simulink model "Discrete_Closed_Loop_Model_74_prelude_simu"  (Simulink 7.8)
settings: Solver=FixedStepDiscrete  StartTime=0.0  StopTime=0.5  FixedStep=dt  RelTol=1e-3
values from neighbouring files (symbols this model uses):
  hc = u(2,k)    [Simul_modele.m]    (also in Simul_modele2.m; Simul_modele3.m; Simul_modele4.m; Simul_modele5.m)
  hcInit = 1e4    (= 10000)    [Simul_modele6.m]    (also in Simul_modele8.m)
  S = sortrows([V' diag(D)],3)    [drawEllipse.m]    (also in tarbouriech04_discret.m = sdpvar(m,m,'diagonal'); tarbouriech05_continu.m = sdpvar(m,m,'diagonal'))
undefined symbols (not defined in the file or in its folder): A_de, A_dx, alpha_0, Az_az, Az_h, Az_q, Az_Va, Az_Vz, B_de, B_dx, Bz_az, Bz_h, Bz_q, Bz_Va, Bz_Vz, C_de, C_dx, cbar, CD_0, CD_alpha, CD_deltae, CI_AltHold, CI_de, CI_dx, CI_FD, CIz_az, CIz_h, CIz_q, CIz_Va, CIz_Vz, CL_alpha, CL_deltae, Cm_0, Cm_alpha, Cm_deltae, Cm_q, Cz_az, Cz_h, Cz_q, Cz_Va, Cz_Vz, D_de, D_dx, delta_e_eq, delta_x_eq, DiscIntNeverNeededParam, dt_dx, Dz_az, Dz_h, Dz_q, Dz_Va, Dz_Vz, g0, h_eq, I_y, K1_intVa, K1_q, K1_Va, K1_Vz, K2_az ... (+21)
settings Model: Creator=David  LastModifiedBy=rpichard  ExtModeAutoUpdateStatusClock=off
settings DataIOCC: LimitDataPoints=off
settings DebuggingCC: SaveWithParameterizedLinksMsg=none  MultiTaskDSMMsg=warning  MultiTaskCondExecSysMsg=none
settings HardwareCC: TargetHWDeviceType=32-bit Generic
settings SFSimCC: SimParseCustomCode=off
settings RTWCC: IncludeERTFirstTime=on
settings CodeAppCC: CustomSymbolStrType=$N$R$M_T
settings GRTTargetCC: TargetFcnLib=ansi_tfl_tmw.mat

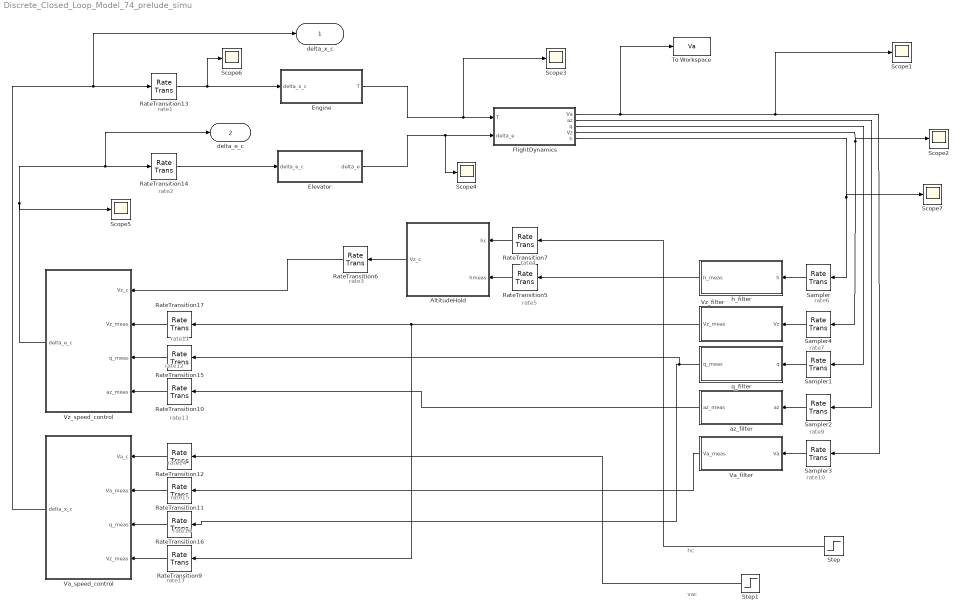
== system Discrete_Closed_Loop_Model_74_prelude_simu ==
  note: rate1
  note: rate2
  note: rate3
  note: rate4
  note: rate5
  note: rate6
  note: rate7
  note: rate9
  note: rate10
  note: rate11
  note: rate12
  note: rate13
  note: rate14
  note: rate15
  note: rate16
  note: rate17
  note: hc
  note: vac
  "AltitudeHold  " : Subsystem
  Elevator : Subsystem
  Engine : Subsystem
  FlightDynamics : Subsystem
  RateTransition{6,10,15,17} (4 alike) : RateTransition  OutPortSampleTime=Ts_K2
  RateTransition{9,11..12,16} (4 alike) : RateTransition  OutPortSampleTime=Ts_K1
  RateTransition13 : RateTransition  X0=delta_x_eq  OutPortSampleTime=dt_dx
  RateTransition14 : RateTransition  X0=delta_e_eq  OutPortSampleTime=dt_de
  RateTransition5 : RateTransition  X0=h_eq  OutPortSampleTime=Ts_h
  RateTransition7 : RateTransition  OutPortSampleTime=Ts_h
  Sampler : RateTransition  X0=h_eq  OutPortSampleTime=Ts_f_h
  Sampler1 : RateTransition  OutPortSampleTime=Ts_f_q
  Sampler2 : RateTransition  OutPortSampleTime=Ts_f_az
  Sampler3 : RateTransition  X0=Va_eq  OutPortSampleTime=Ts_f_Va
      settings: AttributesFormatString=%<Name>
  Sampler4 : RateTransition  OutPortSampleTime=Ts_f_Vz
  Scope{1..7} (7 alike) : Scope
      Scope1 settings: SaveName=ScopeData2
      Scope2 settings: SaveName=ScopeData4
      Scope3 settings: SaveName=ScopeData6
      Scope4 settings: SaveName=ScopeData7
      Scope5 settings: SaveName=ScopeData9
      Scope6 settings: SaveName=ScopeData10
      Scope7 settings: YMin=9990  YMax=10210  SaveName=ScopeData11
  Step : Step  Time=0  Before=hcInit  After=hc  SampleTime=0
  Step1 : Step  Before=235  After=235  SampleTime=0
  To Workspace : ToWorkspace  VariableName=Va  SampleTime=-1  SaveFormat=Array
  Va_filter : Subsystem
  Va_speed_control : Subsystem
  "Vz_filter " : Subsystem
  Vz_speed_control : Subsystem
  az_filter : Subsystem
  "h_filter " : Subsystem
  q_filter : Subsystem
  delta_x_c : Outport
  delta_e_c : Outport  Port=2
  wires:
  Step1/1 -> RateTransition12/1
  FlightDynamics/1(Va) -> Sampler3/1, Scope1/1, To Workspace/1
  FlightDynamics/2(az) -> Sampler2/1
  FlightDynamics/3(q) -> Sampler1/1
  FlightDynamics/4(Vz) -> Sampler4/1, Scope2/1
  Engine/1(T) -> FlightDynamics/1(T), Scope3/1
  Elevator/1(delta_e) -> FlightDynamics/2(delta_e), Scope4/1
  Va_filter/1(Va_meas) -> RateTransition11/1
  "AltitudeHold  "/1(Vz_c) -> RateTransition6/1
  Step/1 -> RateTransition7/1
  FlightDynamics/5(h) -> Sampler/1, Scope7/1
  az_filter/1(az_meas) -> RateTransition10/1
  RateTransition7/1 -> "AltitudeHold  "/1(hc)
  q_filter/1(q_meas) -> RateTransition15/1, RateTransition16/1
  RateTransition10/1 -> Vz_speed_control/4(az_meas)
  RateTransition11/1 -> Va_speed_control/2(Va_meas)
  RateTransition12/1 -> Va_speed_control/1(Va_c)
  Vz_speed_control/1(delta_e_c) -> RateTransition14/1, delta_e_c/1, Scope5/1
  Va_speed_control/1(delta_x_c) -> RateTransition13/1, delta_x_c/1
  RateTransition13/1 -> Engine/1(delta_x_c), Scope6/1
  "h_filter "/1(h_meas) -> RateTransition5/1
  RateTransition15/1 -> Vz_speed_control/3(q_meas)
  RateTransition16/1 -> Va_speed_control/3(q_meas)
  "Vz_filter "/1(Vz_meas) -> RateTransition17/1, RateTransition9/1
  RateTransition9/1 -> Va_speed_control/4(Vz_meas)
  Sampler/1 -> "h_filter "/1(h)
  Sampler4/1 -> "Vz_filter "/1(Vz)
  Sampler1/1 -> q_filter/1(q)
  Sampler2/1 -> az_filter/1(az)
  Sampler3/1 -> Va_filter/1(Va)
  RateTransition5/1 -> "AltitudeHold  "/2(hmeas)
  RateTransition17/1 -> Vz_speed_control/2(Vz_meas)
  RateTransition6/1 -> Vz_speed_control/1(Vz_c)
  RateTransition14/1 -> Elevator/1(delta_e_c)

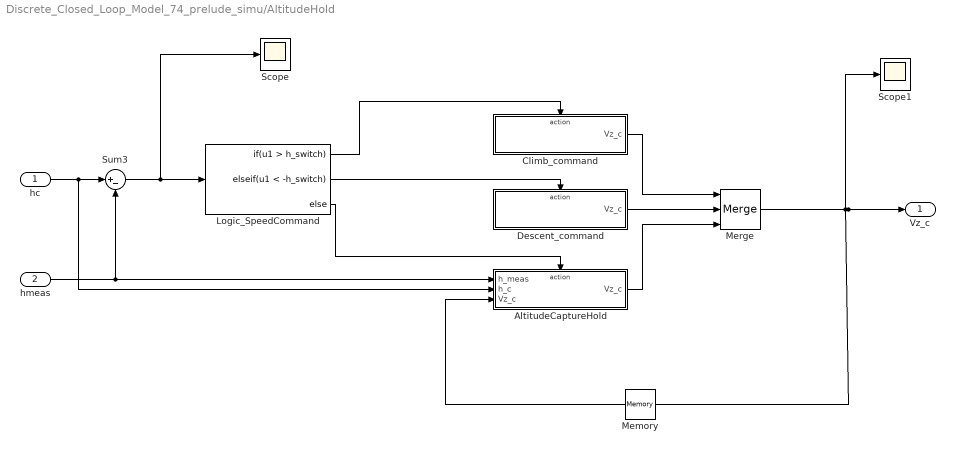
== system Discrete_Closed_Loop_Model_74_prelude_simu/AltitudeHold   ==
  hc : Inport
  hmeas : Inport  Port=2
  AltitudeCaptureHold : Subsystem  TreatAsAtomicUnit=on
  Climb_command : Subsystem  TreatAsAtomicUnit=on
  Descent_command : Subsystem  TreatAsAtomicUnit=on
  Logic_SpeedCommand : If  IfExpression=u1 > h_switch  ElseIfExpressions=u1 < -h_switch
  Memory : Memory  InheritSampleTime=on
  Merge : Merge  Inputs=3
  Scope : Scope
  Scope1 : Scope
      settings: SaveName=ScopeData12
  Sum3 : Sum  Inputs=|+-  SampleTime=Ts_h  OutDataTypeStr=Inherit: Same as first input
  Vz_c : Outport
  wires:
  hc/1 -> AltitudeCaptureHold/2(h_c), Sum3/1
  hmeas/1 -> Sum3/2, AltitudeCaptureHold/1(h_meas)
  Sum3/1 -> Logic_SpeedCommand/1, Scope/1
  Logic_SpeedCommand/1 -> Climb_command/Action
  Logic_SpeedCommand/3 -> AltitudeCaptureHold/Action
  Logic_SpeedCommand/2 -> Descent_command/Action
  Descent_command/1(Vz_c) -> Merge/2
  Climb_command/1(Vz_c) -> Merge/1
  AltitudeCaptureHold/1("Vz_c ") -> Merge/3
  Merge/1 -> Vz_c/1, Memory/1, Scope1/1
  Memory/1 -> AltitudeCaptureHold/3(Vz_c)

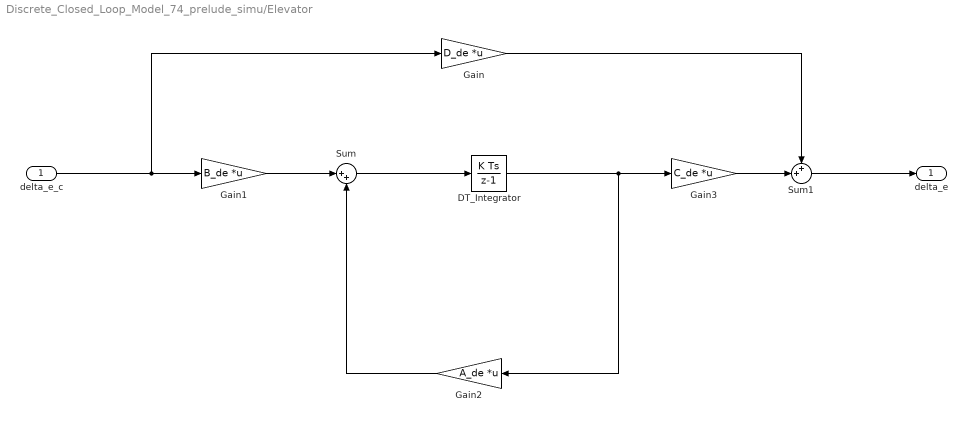
== system Discrete_Closed_Loop_Model_74_prelude_simu/Elevator ==
  delta_e_c : Inport
  DT_Integrator : DiscreteIntegrator  InitialCondition=CI_de  SampleTime=dt_dx  ICPrevOutput=DiscIntNeverNeededParam  ICPrevScaledInput=DiscIntNeverNeededParam
  Gain : Gain  Gain=D_de  Multiplication=Matrix(K*u)  OutDataTypeStr=Inherit: Same as input  ParamDataTypeStr=Inherit: Same as input
  Gain1 : Gain  Gain=B_de  Multiplication=Matrix(K*u)  OutDataTypeStr=Inherit: Same as input  ParamDataTypeStr=Inherit: Same as input
  Gain2 : Gain  Gain=A_de  Multiplication=Matrix(K*u)  OutDataTypeStr=Inherit: Same as input  ParamDataTypeStr=Inherit: Same as input
  Gain3 : Gain  Gain=C_de  Multiplication=Matrix(K*u)  OutDataTypeStr=Inherit: Same as input  ParamDataTypeStr=Inherit: Same as input
  Sum : Sum  Inputs=|++  OutDataTypeStr=Inherit: Same as first input
  Sum1 : Sum  Inputs=++|  OutDataTypeStr=Inherit: Same as first input
  delta_e : Outport
  wires:
  delta_e_c/1 -> Gain/1, Gain1/1
  Sum1/1 -> delta_e/1
  Sum/1 -> DT_Integrator/1
  Gain/1 -> Sum1/1
  Gain1/1 -> Sum/1
  Gain2/1 -> Sum/2
  Gain3/1 -> Sum1/2
  DT_Integrator/1 -> Gain2/1, Gain3/1

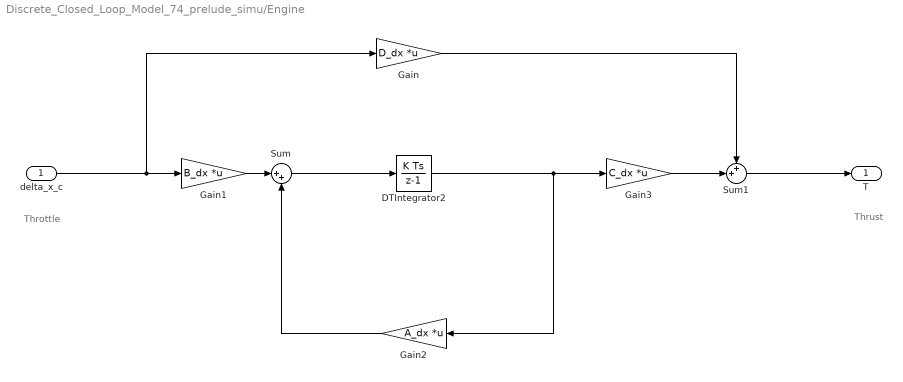
== system Discrete_Closed_Loop_Model_74_prelude_simu/Engine ==
  note: Throttle
  note: Thrust
  delta_x_c : Inport
  DTIntegrator2 : DiscreteIntegrator  InitialCondition=CI_dx  SampleTime=dt_dx  ICPrevOutput=DiscIntNeverNeededParam  ICPrevScaledInput=DiscIntNeverNeededParam
  Gain : Gain  Gain=D_dx  Multiplication=Matrix(K*u)  OutDataTypeStr=Inherit: Same as input  ParamDataTypeStr=Inherit: Same as input
  Gain1 : Gain  Gain=B_dx  Multiplication=Matrix(K*u)  OutDataTypeStr=Inherit: Same as input  ParamDataTypeStr=Inherit: Same as input
  Gain2 : Gain  Gain=A_dx  Multiplication=Matrix(K*u)  OutDataTypeStr=Inherit: Same as input  ParamDataTypeStr=Inherit: Same as input
  Gain3 : Gain  Gain=C_dx  Multiplication=Matrix(K*u)  OutDataTypeStr=Inherit: Same as input  ParamDataTypeStr=Inherit: Same as input
  Sum : Sum  Inputs=|++  OutDataTypeStr=Inherit: Same as first input
  Sum1 : Sum  Inputs=++|  OutDataTypeStr=Inherit: Same as first input
  T : Outport
  wires:
  delta_x_c/1 -> Gain/1, Gain1/1
  Sum1/1 -> T/1
  DTIntegrator2/1 -> Gain2/1, Gain3/1
  Sum/1 -> DTIntegrator2/1
  Gain/1 -> Sum1/1
  Gain1/1 -> Sum/1
  Gain2/1 -> Sum/2
  Gain3/1 -> Sum1/2

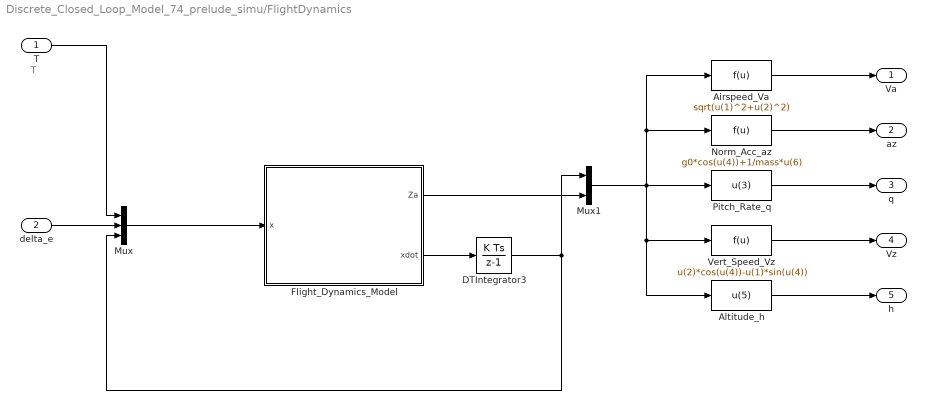
== system Discrete_Closed_Loop_Model_74_prelude_simu/FlightDynamics ==
  note: T
  T : Inport
  delta_e : Inport  Port=2
  "Airspeed_Va  " : Fcn  Expr=sqrt(u(1)^2+u(2)^2)
  Altitude_h : Fcn  Expr=u(5)
  DTIntegrator3 : DiscreteIntegrator  InitialCondition=CI_FD  SampleTime=dt_dx  ICPrevOutput=DiscIntNeverNeededParam  ICPrevScaledInput=DiscIntNeverNeededParam
  Flight_Dynamics_Model : Subsystem
  Mux : Mux  Inputs=3
  Mux1 : Mux  Inputs=2
  "Norm_Acc_az  " : Fcn  Expr=g0*cos(u(4))+1/mass*u(6)
  "Pitch_Rate_q " : Fcn  Expr=u(3)
  Vert_Speed_Vz : Fcn  Expr=u(2)*cos(u(4))-u(1)*sin(u(4))
  Va : Outport
  az : Outport  Port=2
  q : Outport  Port=3
  Vz : Outport  Port=4
  h : Outport  Port=5
  wires:
  delta_e/1 -> Mux/2
  DTIntegrator3/1 -> Mux/3, Mux1/1
  T/1 -> Mux/1
  Mux/1 -> Flight_Dynamics_Model/1(x)
  Flight_Dynamics_Model/2(xdot) -> DTIntegrator3/1
  Altitude_h/1 -> h/1
  Vert_Speed_Vz/1 -> Vz/1
  "Pitch_Rate_q "/1 -> q/1
  "Norm_Acc_az  "/1 -> az/1
  "Airspeed_Va  "/1 -> Va/1
  Flight_Dynamics_Model/1(Za) -> Mux1/2
  Mux1/1 -> "Pitch_Rate_q "/1, "Norm_Acc_az  "/1, "Airspeed_Va  "/1, Vert_Speed_Vz/1, Altitude_h/1

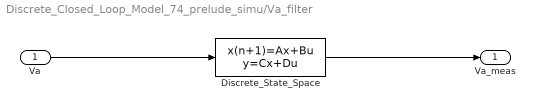
== system Discrete_Closed_Loop_Model_74_prelude_simu/Va_filter ==
  Va : Inport
  Discrete_State_Space : DiscreteStateSpace  A=Az_Va  B=Bz_Va  C=Cz_Va  D=Dz_Va  X0=CIz_Va  SampleTime=Ts_f_Va
  Va_meas : Outport
  wires:
  Discrete_State_Space/1 -> Va_meas/1
  Va/1 -> Discrete_State_Space/1

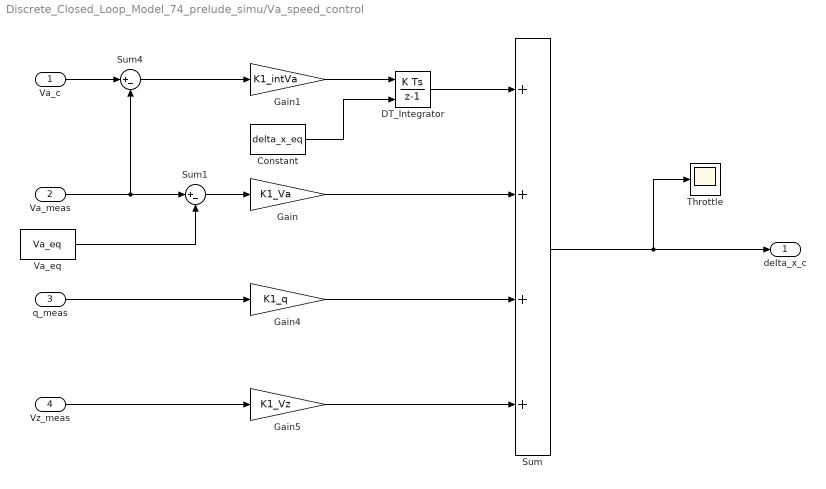
== system Discrete_Closed_Loop_Model_74_prelude_simu/Va_speed_control ==
  Va_c : Inport
  Va_meas : Inport  Port=2
  q_meas : Inport  Port=3
  Vz_meas : Inport  Port=4
  Constant : Constant  Value=delta_x_eq  SampleTime=Ts_K1
  DT_Integrator : DiscreteIntegrator  InitialConditionSource=external  SampleTime=Ts_K1  ICPrevOutput=DiscIntNeverNeededParam  ICPrevScaledInput=DiscIntNeverNeededParam
  Gain : Gain  Gain=K1_Va  OutDataTypeStr=Inherit: Same as input  ParamDataTypeStr=Inherit: Same as input
  Gain1 : Gain  Gain=K1_intVa  OutDataTypeStr=Inherit: Same as input  ParamDataTypeStr=Inherit: Same as input
  Gain4 : Gain  Gain=K1_q  OutDataTypeStr=Inherit: Same as input  ParamDataTypeStr=Inherit: Same as input
  Gain5 : Gain  Gain=K1_Vz  OutDataTypeStr=Inherit: Same as input  ParamDataTypeStr=Inherit: Same as input
  Sum : Sum  Inputs=++++  SampleTime=Ts_K1  OutDataTypeStr=Inherit: Same as first input
  Sum1 : Sum  Inputs=|+-  SampleTime=Ts_K1  OutDataTypeStr=Inherit: Same as first input
  Sum4 : Sum  Inputs=|+-  SampleTime=Ts_K1  OutDataTypeStr=Inherit: Same as first input
  Throttle : Scope
      settings: YMin=10094  YMax=10100.5  SaveName=ScopeData5  DataFormat=Array
  Va_eq : Constant  Value=Va_eq  SampleTime=Ts_K1
  delta_x_c : Outport
  wires:
  Va_meas/1 -> Sum1/1, Sum4/2
  Sum1/1 -> Gain/1
  Gain/1 -> Sum/2
  Va_c/1 -> Sum4/1
  Gain1/1 -> DT_Integrator/1
  q_meas/1 -> Gain4/1
  Vz_meas/1 -> Gain5/1
  Gain4/1 -> Sum/3
  Gain5/1 -> Sum/4
  Sum/1 -> Throttle/1, delta_x_c/1
  Constant/1 -> DT_Integrator/2
  Va_eq/1 -> Sum1/2
  Sum4/1 -> Gain1/1
  DT_Integrator/1 -> Sum/1

== system Discrete_Closed_Loop_Model_74_prelude_simu/Vz_filter  ==
  Vz : Inport
  Discrete_State_Space : DiscreteStateSpace  A=Az_Vz  B=Bz_Vz  C=Cz_Vz  D=Dz_Vz  X0=CIz_Vz  SampleTime=Ts_f_Vz
  Vz_meas : Outport
  wires:
  Discrete_State_Space/1 -> Vz_meas/1
  Vz/1 -> Discrete_State_Space/1

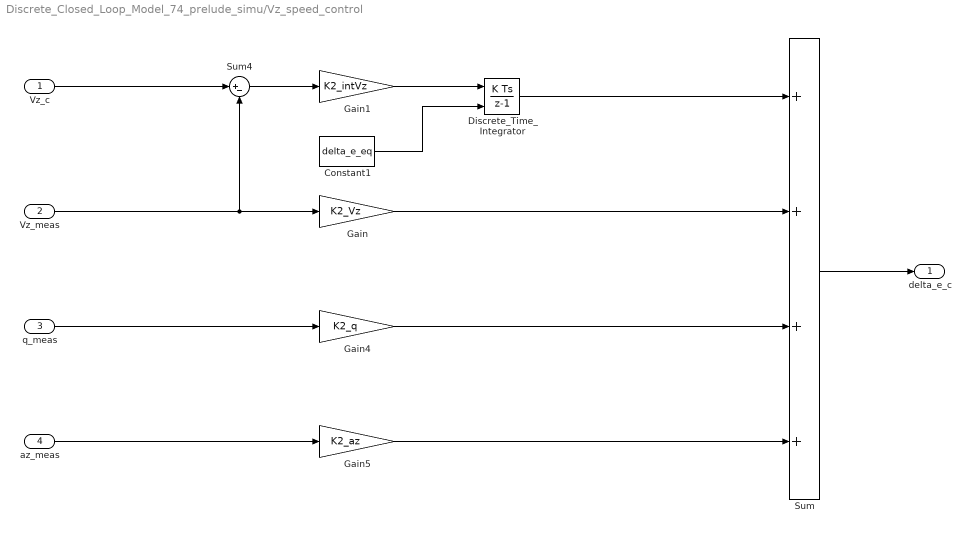
== system Discrete_Closed_Loop_Model_74_prelude_simu/Vz_speed_control ==
  Vz_c : Inport
  Vz_meas : Inport  Port=2
  q_meas : Inport  Port=3
  az_meas : Inport  Port=4
  Constant1 : Constant  Value=delta_e_eq  SampleTime=Ts_K2
  Discrete_Time_Integrator : DiscreteIntegrator  InitialConditionSource=external  SampleTime=Ts_K2  ICPrevOutput=DiscIntNeverNeededParam  ICPrevScaledInput=DiscIntNeverNeededParam
  Gain : Gain  Gain=K2_Vz  OutDataTypeStr=Inherit: Same as input  ParamDataTypeStr=Inherit: Same as input
  Gain1 : Gain  Gain=K2_intVz  OutDataTypeStr=Inherit: Same as input  ParamDataTypeStr=Inherit: Same as input
  Gain4 : Gain  Gain=K2_q  OutDataTypeStr=Inherit: Same as input  ParamDataTypeStr=Inherit: Same as input
  Gain5 : Gain  Gain=K2_az  OutDataTypeStr=Inherit: Same as input  ParamDataTypeStr=Inherit: Same as input
  Sum : Sum  Inputs=++++  SampleTime=Ts_K2  OutDataTypeStr=Inherit: Same as first input
  Sum4 : Sum  Inputs=|+-  OutDataTypeStr=Inherit: Same as first input
  delta_e_c : Outport
  wires:
  Vz_meas/1 -> Sum4/2, Gain/1
  Gain/1 -> Sum/2
  Vz_c/1 -> Sum4/1
  Gain1/1 -> Discrete_Time_Integrator/1
  q_meas/1 -> Gain4/1
  az_meas/1 -> Gain5/1
  Gain4/1 -> Sum/3
  Gain5/1 -> Sum/4
  Sum/1 -> delta_e_c/1
  Sum4/1 -> Gain1/1
  Discrete_Time_Integrator/1 -> Sum/1
  Constant1/1 -> Discrete_Time_Integrator/2

== system Discrete_Closed_Loop_Model_74_prelude_simu/az_filter ==
  az : Inport
  Discrete_State_Space : DiscreteStateSpace  A=Az_az  B=Bz_az  C=Cz_az  D=Dz_az  X0=CIz_az  SampleTime=Ts_f_az
  az_meas : Outport
  wires:
  Discrete_State_Space/1 -> az_meas/1
  az/1 -> Discrete_State_Space/1

== system Discrete_Closed_Loop_Model_74_prelude_simu/h_filter  ==
  h : Inport
  Discrete_State_Space : DiscreteStateSpace  A=Az_h  B=Bz_h  C=Cz_h  D=Dz_h  X0=CIz_h  SampleTime=Ts_f_h
  h_meas : Outport
  wires:
  Discrete_State_Space/1 -> h_meas/1
  h/1 -> Discrete_State_Space/1

== system Discrete_Closed_Loop_Model_74_prelude_simu/q_filter ==
  q : Inport
  Discrete_State_Space : DiscreteStateSpace  A=Az_q  B=Bz_q  C=Cz_q  D=Dz_q  X0=CIz_q  SampleTime=Ts_f_q
  q_meas : Outport
  wires:
  Discrete_State_Space/1 -> q_meas/1
  q/1 -> Discrete_State_Space/1

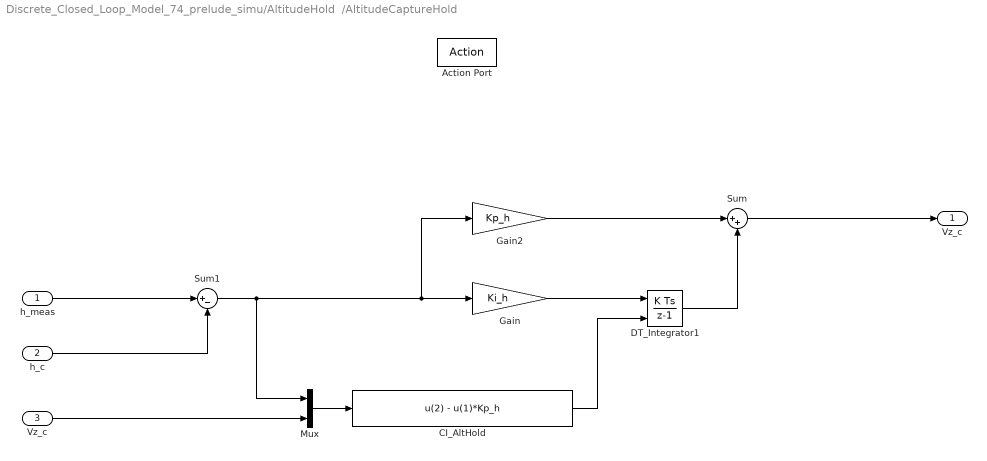
== system Discrete_Closed_Loop_Model_74_prelude_simu/AltitudeHold  /AltitudeCaptureHold ==
  h_meas : Inport
  h_c : Inport  Port=2
  Vz_c : Inport  Port=3
  Action Port : ActionPort  InitializeStates=reset  ActionType=else
  CI_AltHold : Fcn  Expr=u(2) - u(1)*Kp_h
  DT_Integrator1 : DiscreteIntegrator  InitialConditionSource=external  InitialCondition=CI_AltHold  SampleTime=Ts_h  ICPrevOutput=DiscIntNeverNeededParam  ICPrevScaledInput=DiscIntNeverNeededParam
  Gain : Gain  Gain=Ki_h  OutDataTypeStr=Inherit: Same as input  ParamDataTypeStr=Inherit: Same as input
  Gain2 : Gain  Gain=Kp_h  OutDataTypeStr=Inherit: Same as input  ParamDataTypeStr=Inherit: Same as input
  Mux : Mux  Inputs=2
  Sum : Sum  Inputs=|++  OutDataTypeStr=Inherit: Same as first input
  Sum1 : Sum  Inputs=|+-  OutDataTypeStr=Inherit: Same as first input
  "Vz_c " : Outport
  wires:
  Gain/1 -> DT_Integrator1/1
  Gain2/1 -> Sum/1
  h_meas/1 -> Sum1/1
  CI_AltHold/1 -> DT_Integrator1/2
  Sum/1 -> "Vz_c "/1
  Sum1/1 -> Mux/1, Gain/1, Gain2/1
  h_c/1 -> Sum1/2
  DT_Integrator1/1 -> Sum/2
  Mux/1 -> CI_AltHold/1
  Vz_c/1 -> Mux/2

== system Discrete_Closed_Loop_Model_74_prelude_simu/AltitudeHold  /Climb_command ==
  Action Port : ActionPort  ActionType=then
  h_switch2 : Constant  Value=Vz_c  SampleTime=Ts_h
  Vz_c : Outport
  wires:
  h_switch2/1 -> Vz_c/1

== system Discrete_Closed_Loop_Model_74_prelude_simu/AltitudeHold  /Descent_command ==
  Action Port : ActionPort  InitializeStates=reset  ActionType=elseif
  h_switch4 : Constant  Value=-Vz_c  SampleTime=Ts_h
  Vz_c : Outport
  wires:
  h_switch4/1 -> Vz_c/1

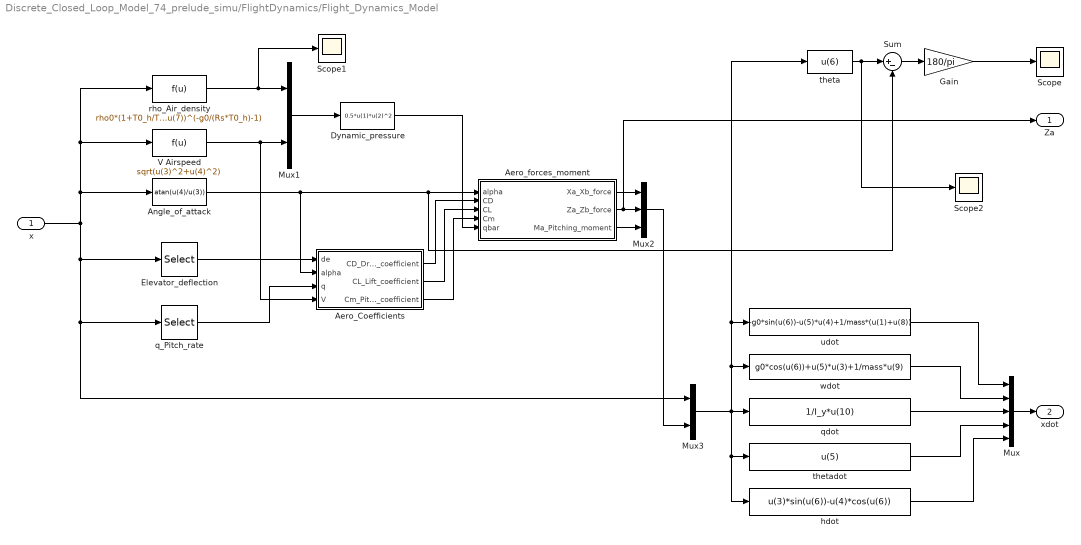
== system Discrete_Closed_Loop_Model_74_prelude_simu/FlightDynamics/Flight_Dynamics_Model ==
  x : Inport
  Aero_Coefficients : Subsystem
  Aero_forces_moment : Subsystem
  Angle_of_attack : Fcn  Expr=atan(u(4)/u(3))
  Dynamic_pressure : Fcn  Expr=0.5*u(1)*u(2)^2
  Elevator_deflection : Selector  InputPortWidth=7  IndexOptions=Index vector (dialog)  Indices=[2]  OutputSizes=1
  Gain : Gain  Gain=180/pi  OutDataTypeStr=Inherit: Same as input  ParamDataTypeStr=Inherit: Same as input
  Mux : Mux  Inputs=5
  Mux1 : Mux  Inputs=2
  Mux2 : Mux  Inputs=3
  Mux3 : Mux  Inputs=2
  Scope : Scope
      settings: YMin=-0.001  YMax=0.011
  Scope1 : Scope
      settings: YMin=-0.001  YMax=0.011  SaveName=ScopeData3
  Scope2 : Scope
      settings: YMin=-0.001  YMax=0.011  SaveName=ScopeData8
  Sum : Sum  Inputs=|+-  OutDataTypeStr=Inherit: Same as first input
  V Airspeed : Fcn  Expr=sqrt(u(3)^2+u(4)^2)
  hdot : Fcn  Expr=u(3)*sin(u(6))-u(4)*cos(u(6))
  q_Pitch_rate : Selector  InputPortWidth=7  IndexOptions=Index vector (dialog)  Indices=[5]  OutputSizes=1
  qdot : Fcn  Expr=1/I_y*u(10)
  rho_Air_density : Fcn  Expr=rho0*(1+T0_h/T0_0*u(7))^(-g0/(Rs*T0_h)-1)
  theta : Fcn  Expr=u(6)
  thetadot : Fcn  Expr=u(5)
  udot : Fcn  Expr=-g0*sin(u(6))-u(5)*u(4)+1/mass*(u(1)+u(8))
  wdot : Fcn  Expr=g0*cos(u(6))+u(5)*u(3)+1/mass*u(9)
  Za : Outport
  xdot : Outport  Port=2
  wires:
  udot/1 -> Mux/1
  wdot/1 -> Mux/2
  qdot/1 -> Mux/3
  thetadot/1 -> Mux/4
  hdot/1 -> Mux/5
  Mux/1 -> xdot/1
  x/1 -> Elevator_deflection/1, q_Pitch_rate/1, Mux3/1, rho_Air_density/1, V Airspeed/1, Angle_of_attack/1
  rho_Air_density/1 -> Scope1/1, Mux1/1
  V Airspeed/1 -> Mux1/2, Aero_Coefficients/4(V)
  Mux1/1 -> Dynamic_pressure/1
  Elevator_deflection/1 -> Aero_Coefficients/1(de)
  Angle_of_attack/1 -> Aero_forces_moment/1(alpha), Sum/2, Aero_Coefficients/2(alpha)
  q_Pitch_rate/1 -> Aero_Coefficients/3(q)
  Dynamic_pressure/1 -> Aero_forces_moment/5(qbar)
  Aero_Coefficients/1(CD_Drag_coefficient) -> Aero_forces_moment/2(CD)
  Aero_Coefficients/2(CL_Lift_coefficient) -> Aero_forces_moment/3(CL)
  Aero_Coefficients/3(Cm_Pitching_coefficient) -> Aero_forces_moment/4(Cm)
  Aero_forces_moment/1("Xa_Xb_force ") -> Mux2/1
  Aero_forces_moment/2(Za_Zb_force) -> Za/1, Mux2/2
  Aero_forces_moment/3(Ma_Pitching_moment) -> Mux2/3
  Mux2/1 -> Mux3/2
  Mux3/1 -> theta/1, udot/1, wdot/1, qdot/1, thetadot/1, hdot/1
  Sum/1 -> Gain/1
  theta/1 -> Sum/1, Scope2/1
  Gain/1 -> Scope/1

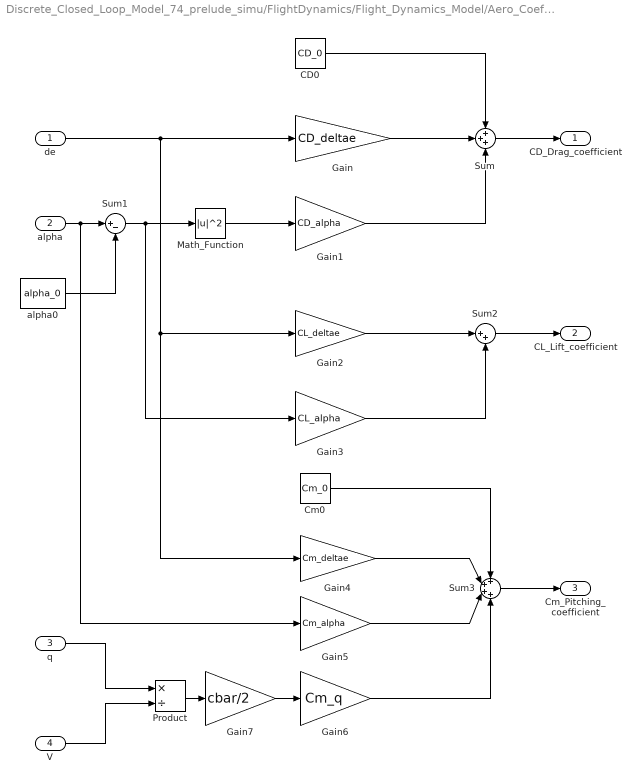
== system Discrete_Closed_Loop_Model_74_prelude_simu/FlightDynamics/Flight_Dynamics_Model/Aero_Coefficients ==
  de : Inport
  alpha : Inport  Port=2
  q : Inport  Port=3
  V : Inport  Port=4
  CD0 : Constant  Value=CD_0
  Cm0 : Constant  Value=Cm_0
  Gain : Gain  Gain=CD_deltae  OutDataTypeStr=Inherit: Same as input  ParamDataTypeStr=Inherit: Same as input
  Gain1 : Gain  Gain=CD_alpha  OutDataTypeStr=Inherit: Same as input  ParamDataTypeStr=Inherit: Same as input
  Gain2 : Gain  Gain=CL_deltae  OutDataTypeStr=Inherit: Same as input  ParamDataTypeStr=Inherit: Same as input
  Gain3 : Gain  Gain=CL_alpha  OutDataTypeStr=Inherit: Same as input  ParamDataTypeStr=Inherit: Same as input
  Gain4 : Gain  Gain=Cm_deltae  OutDataTypeStr=Inherit: Same as input  ParamDataTypeStr=Inherit: Same as input
  Gain5 : Gain  Gain=Cm_alpha  OutDataTypeStr=Inherit: Same as input  ParamDataTypeStr=Inherit: Same as input
  Gain6 : Gain  Gain=Cm_q  OutDataTypeStr=Inherit: Same as input  ParamDataTypeStr=Inherit: Same as input
  Gain7 : Gain  Gain=cbar/2  OutDataTypeStr=Inherit: Same as input  ParamDataTypeStr=Inherit: Same as input
  Math_Function : Math  Operator=magnitude^2  SaturateOnIntegerOverflow=on
  Product : Product  Inputs=*/  RndMeth=Zero  OutDataTypeStr=Inherit: Same as first input
  Sum : Sum  Inputs=+++  OutDataTypeStr=Inherit: Same as first input
  Sum1 : Sum  Inputs=|+-  OutDataTypeStr=Inherit: Same as first input
  Sum2 : Sum  Inputs=|++  OutDataTypeStr=Inherit: Same as first input
  Sum3 : Sum  Inputs=++++  OutDataTypeStr=Inherit: Same as first input
  alpha0 : Constant  Value=alpha_0
  CD_Drag_coefficient : Outport
  CL_Lift_coefficient : Outport  Port=2
  Cm_Pitching_coefficient : Outport  Port=3
  wires:
  de/1 -> Gain/1, Gain2/1, Gain4/1
  CD0/1 -> Sum/1
  Gain/1 -> Sum/2
  Gain1/1 -> Sum/3
  Sum/1 -> CD_Drag_coefficient/1
  alpha/1 -> Sum1/1, Gain5/1
  alpha0/1 -> Sum1/2
  Sum1/1 -> Math_Function/1, Gain3/1
  Math_Function/1 -> Gain1/1
  Gain3/1 -> Sum2/2
  Sum2/1 -> CL_Lift_coefficient/1
  Gain2/1 -> Sum2/1
  Cm0/1 -> Sum3/1
  Gain4/1 -> Sum3/2
  Gain5/1 -> Sum3/3
  Sum3/1 -> Cm_Pitching_coefficient/1
  Gain6/1 -> Sum3/4
  q/1 -> Product/1
  V/1 -> Product/2
  Product/1 -> Gain7/1
  Gain7/1 -> Gain6/1

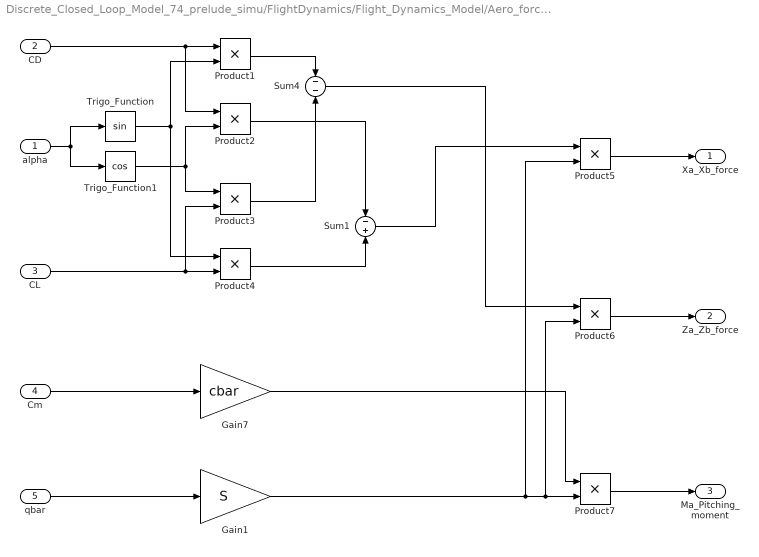
== system Discrete_Closed_Loop_Model_74_prelude_simu/FlightDynamics/Flight_Dynamics_Model/Aero_forces_moment ==
  alpha : Inport
  CD : Inport  Port=2
  CL : Inport  Port=3
  Cm : Inport  Port=4
  qbar : Inport  Port=5
  Gain1 : Gain  Gain=S  OutDataTypeStr=Inherit: Same as input  ParamDataTypeStr=Inherit: Same as input
  Gain7 : Gain  Gain=cbar  OutDataTypeStr=Inherit: Same as input  ParamDataTypeStr=Inherit: Same as input
  Product{1..7} (7 alike) : Product  RndMeth=Zero  OutDataTypeStr=Inherit: Same as first input
  Sum1 : Sum  Inputs=-+  OutDataTypeStr=Inherit: Same as first input
  Sum4 : Sum  Inputs=--  OutDataTypeStr=Inherit: Same as first input
  Trigo_Function : Trigonometry
  Trigo_Function1 : Trigonometry  Operator=cos
  "Xa_Xb_force " : Outport
  Za_Zb_force : Outport  Port=2
  Ma_Pitching_moment : Outport  Port=3
  wires:
  Product5/1 -> "Xa_Xb_force "/1
  Product6/1 -> Za_Zb_force/1
  Product7/1 -> Ma_Pitching_moment/1
  alpha/1 -> Trigo_Function/1, Trigo_Function1/1
  CD/1 -> Product1/1, Product2/1
  Trigo_Function/1 -> Product1/2, Product4/1
  Trigo_Function1/1 -> Product2/2, Product3/1
  CL/1 -> Product4/2, Product3/2
  Product4/1 -> Sum1/2
  Product2/1 -> Sum1/1
  Product1/1 -> Sum4/1
  Product3/1 -> Sum4/2
  Sum4/1 -> Product6/1
  Cm/1 -> Gain7/1
  Gain7/1 -> Product7/1
  Sum1/1 -> Product5/1
  qbar/1 -> Gain1/1
  Gain1/1 -> Product7/2, Product6/2, Product5/2
